simulink model "sf_countflowers"  (R2021a)
settings: Solver=FixedStepDiscrete  StartTime=0.0  StopTime=fisheririsInput.time(end)  FixedStep=1  RelTol=1e-3  EnableMultiTasking=on
settings Model: Creator=The MathWorks, Inc.  LastModifiedBy=The MathWorks, Inc.
settings SolverCC: AlgebraicLoopSolver=TrustRegion  AutoInsertRateTranBlk=on
settings DataIOCC: ExternalInput=fisheririsInput  LimitDataPoints=on  LoadExternalInput=on  SaveOutput=off  DSMLogging=off  SaveTime=off  ReturnWorkspaceOutputs=off
settings OptimizationCC: LifeSpan=inf
settings DebuggingCC: AllowSymbolicDim=off  SFUnexpectedBacktrackingDiag=warning  SFNoUnconditionalDefaultTransitionDiag=warning  SFExecutionAtInitializationDiag=none  SFMachineParentedDataDiag=warning  ArithmeticOperatorsInVariantConditions=warning
settings SFSimCC: SimUseLocalCustomCode=off
settings RTWCC: GenerateReport=on  RTWUseLocalCustomCode=off  LaunchReport=on
settings CodeAppCC: StateflowObjectComments=on
settings GRTTargetCC: TargetLangStandard=C89/C90 (ANSI)
settings ConfigComp: CovMetricSettings=dw  CovSaveCumulativeToWorkspaceVar=on  CovSaveSingleToWorkspaceVar=on  CovExternalEMLEnable=off  CovSFcnEnable=off

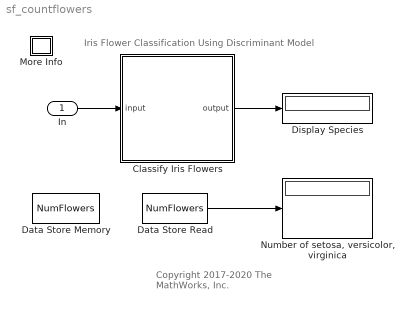
== system sf_countflowers ==
  note: Iris Flower Classification Using Discriminant Model
  note: Copyright 2017-2020 The MathWorks, Inc.
  In : Inport  PortDimensions=[4]
  Classify Iris Flowers : Stateflow chart  TreatAsAtomicUnit=on
  Data Store Memory : DataStoreMemory  DataStoreName=NumFlowers  InitialValue=[0 0 0]  ShowAdditionalParam=off  OutDataTypeStr=double
  Data Store Read : DataStoreRead  DataStoreName=NumFlowers  IndexOptions=Index vector (dialog)  Indices=1  OutputSizes=1
  Display Species : Display
  More Info : Subsystem
      settings: OpenFcn=showExample('stats/PredictClassLabelsUsingStateflowExample')
      mask Display: disp('?')
  "Number of setosa, versicolor, virginica " : Display
  wires:
  In/1 -> Classify Iris Flowers/1(input)
  Data Store Read/1 -> "Number of setosa, versicolor, virginica "/1
  Classify Iris Flowers/1(output) -> Display Species/1

== system sf_countflowers/More Info ==

== stateflow chart sf_countflowers/Classify Iris Flowers ==
  (default) -> (junction 40) : {output = mypredict(input);}
  (junction 40) -> (junction 41) [order 1] : [output == Setosa]
  (junction 40) -> (junction 42) [order 2]
  (junction 41) -> (junction 46) : {NumFlowers(1) = NumFlowers(1) + 1;}
  (junction 42) -> (junction 43) [order 1] : [output == Versicolor]
  (junction 42) -> (junction 44) [order 2] : {NumFlowers(3) = NumFlowers(3) + 1;}
  (junction 43) -> (junction 45) : {NumFlowers(2) = NumFlowers(2) + 1;}
  (junction 45) -> (junction 44)
  (junction 46) -> (junction 45)
  (junction 44) -> (junction 47)
  data: label function_output Enum: IrisSpecies size=[1,1]; X function_input; input input size=[1,4]; NumFlowers data_store_memory; output output size=[1,1]
  function label  = mypredict(X):
    | function label  = mypredict(X) %#codegen
    | %MYPREDICT Predict species of iris flowers using discriminant model
    | %   mypredict predicts species of iris flowers using the compact
    | %   discriminant model in the file DiscrIris.mat. Rows of X correspond to
    | %   observations and columns correspond to predictor variables. label is
    | %   the predicted species.
    | mdl = loadLearnerForCoder('DiscrIris');
    | labelTemp = predict(mdl,X);
    | label = IrisSpecies(labelTemp);
    | end
